simulink model "EdgeDetectionPictureDSK6416"  (Simulink 6.5)
settings: Solver=FixedStepDiscrete  StartTime=0.0  StopTime=inf  RelTol=1e-3
libraries: rtdxBlocks x2, c6000tgtpreflib x1, vipanalysis x1, vipconversions x1
settings Model: Creator=greith  LastModifiedBy=jacobf  ProdHWDeviceType=TI C6000
settings SolverCC: PositivePriorityOrder=on
settings DataIOCC: SaveOutput=off  SaveTime=off
settings OptimizationCC: OptimizeModelRefInitCode=on
settings HardwareCC: ProdBitPerLong=40  ProdIntDivRoundTo=Zero  ProdEndianess=LittleEndian  ProdHWDeviceType=TI C6000
settings RTWCC: SystemTargetFile=ti_c6000_ert.tlc  GenCodeOnly=on  TemplateMakefile=ti_c6000_ert.tmf  Description=Embedded Target for TI C6000 DSP (ERT)  ProcessScript=ti_c6000_ert_make_rtw_hook
settings CodeAppCC: IgnoreCustomStorageClasses=off
settings C6000ERTTargetCC: TargetFcnLib=ansi_tfl_tmw.mat  GenFloatMathFcnCalls=ANSI_C  UtilityFuncGeneration=Auto  GenerateFullHeader=on  GenerateSampleERTMain=off  GenerateTestInterfaces=off  IsPILTarget=off  ModelReferenceCompliant=on  IncludeMdlTerminateFcn=on  CombineOutputUpdateFcns=on  SuppressErrorStatus=off  IncludeFileDelimiter=Auto  ERTCustomFileBanners=on  SupportAbsoluteTime=on  LogVarNameModifier=rt_  MatFileLogging=off  MultiInstanceERTCode=off  SupportNonFinite=on  SupportComplex=on  PurelyIntegerCode=off  SupportContinuousTime=off  SupportNonInlinedSFcns=off  EnableShiftOperators=on  ParenthesesLevel=Nominal  GenerateErtSFunction=off  GenerateASAP2=off  ExtMode=off  ExtModeTransport=0  ExtModeStaticAlloc=off  ExtModeStaticAllocSize=1000000  ExtModeTesting=off  ExtModeMexFile=ext_comm  InlinedParameterPlacement=NonHierarchical  TargetOS=BareBoardExample  MultiInstanceErrorCode=Error  RateGroupingCode=on  RootIOFormat=Individual arguments  RTWCAPISignals=off  RTWCAPIParams=off  RTWCAPIStates=off  ERTSrcFileBannerTemplate=ert_code_template.cgt  ERTHdrFileBannerTemplate=ert_code_template.cgt  ERTDataSrcFileTemplate=ert_code_template.cgt  ERTDataHdrFileTemplate=ert_code_template.cgt  ERTCustomFileTemplate=example_file_process.tlc  ModuleNamingRule=Unspecified  SignalDisplayLevel=10  ParamTuneLevel=10  GlobalDataDefinition=Auto  DataDefinitionFile=global.c  GlobalDataReference=Auto  DataReferenceFile=global.h  GRTInterface=off  EnableUserReplacementTypes=off  MemSecPackage=--- None ---  MemSecDataConstants=Default  MemSecDataIO=Default  MemSecDataInternal=Default  MemSecDataParameters=Default  MemSecFuncInitTerm=Default  MemSecFuncExecute=Default  exportCCSObj=on  ccsObjName=CCS_Obj  useDSPBIOS=on  ProfileGenCode=off  InlineDSPBlks=on  FPopt=off  memModel=Far_Aggregate  optLevel=Function(-o2)  CompilerVerbosity=Quiet  InterruptThreshOnC6x=off  SymbolicDebugOnC6x=off  RetainAsmFiles=off  RetainObjFiles=on  CreateMapFile=on  UserStackSize=8192  c6000BuildAction=Build  OverrunAction=None  OverrunNotificationMethod=Turn_on_LEDs

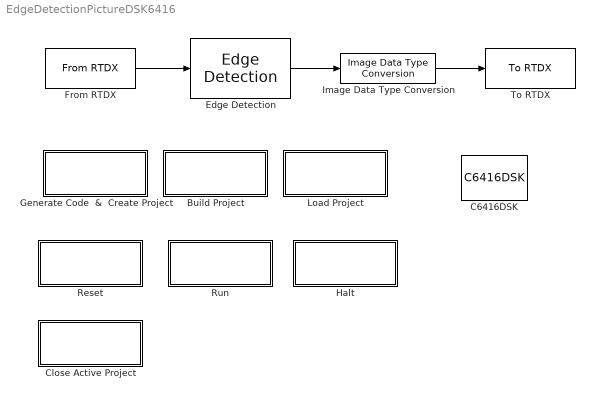
== system EdgeDetectionPictureDSK6416 ==
  Build Project : Subsystem
      settings: OpenFcn=CCS_Obj.build;
      mask Display: disp('Build\nProject')
  C6416DSK : c6000tgtpreflib/C6416DSK  Tag=C6000 TARGET PREFERENCES BLOCK  SystemSampleTime=-1
  Close Active Project : Subsystem
      settings: OpenFcn=close(CCS_Obj,[],'project')
      mask Display: disp('Close Active Project')
  Edge Detection : vipanalysis/Edge Detection  DialogController=vipDDGCreate  DialogControllerArgs=DataTag1  method=Sobel  outputType=Binary image  userDefinedThreshold=off  thresholdSource=Input port  threshold=20  thresholdTuning=1  edgeThinning=off  threshold_canny=[0.25 0.60]  autoPercent=70  sigma=1  prodOutputMode=Binary point scaling  prodOutputWordLength=32  prodOutputFracLength=8  roundingMode=Floor  overflowMode=off
  From RTDX : rtdxBlocks/From RTDX  channelNameStr=inputimage  isBlocking=on  icMaskVar=0  Ts=-1  dims=[65 309]  isFrame=off  dType=uint8  isChannelEnabled=on  isHighSpeedRTDXUsed=on
  Generate Code  &  Create Project : Subsystem
      settings: OpenFcn=make_rtw;
      mask Display: disp('Generate Code\n & \nCreate Project')
  Halt : Subsystem
      settings: OpenFcn=CCS_Obj.halt;
      mask Display: disp('Halt')
  Image Data Type Conversion : vipconversions/Image Data Type Conversion  outDT=uint8  isSigned=on  wordLen=16  numFracBits=0
  Load Project : Subsystem
      settings: OpenFcn=CCS_Obj.load([pwd,'\',bdroot,'_c6000_rtw\', bdroot, '.out'])
      mask Display: disp('Load\nProject')
  Reset : Subsystem
      settings: OpenFcn=CCS_Obj.reset;
      mask Display: disp('Reset')
  Run : Subsystem
      settings: OpenFcn=CCS_Obj.run;
      mask Display: disp('Run')
  To RTDX : rtdxBlocks/To RTDX  channelNameStr=outputimage  isBlocking=on  isChannelEnabled=on
  wires:
  Edge Detection/1 -> Image Data Type Conversion/1
  From RTDX/1 -> Edge Detection/1
  Image Data Type Conversion/1 -> To RTDX/1

== system EdgeDetectionPictureDSK6416/Build Project ==

== system EdgeDetectionPictureDSK6416/Close Active Project ==

== system EdgeDetectionPictureDSK6416/Generate Code  &  Create Project ==

== system EdgeDetectionPictureDSK6416/Halt ==

== system EdgeDetectionPictureDSK6416/Load Project ==

== system EdgeDetectionPictureDSK6416/Reset ==

== system EdgeDetectionPictureDSK6416/Run ==
